simulink model "c00015M_harness"  (R2018a)
settings: Solver=FixedStepAuto  StartTime=0.0  StopTime=300  FixedStep=0.1  RelTol=1e-3
undefined symbols (not defined in the file): A1, hmax, PriorityTank, R1, R2, sigbuilder_block, TempThreshold
(part 1 of 33)
settings Model: Creator=aarrieta  LastModifiedBy=umarkiegi

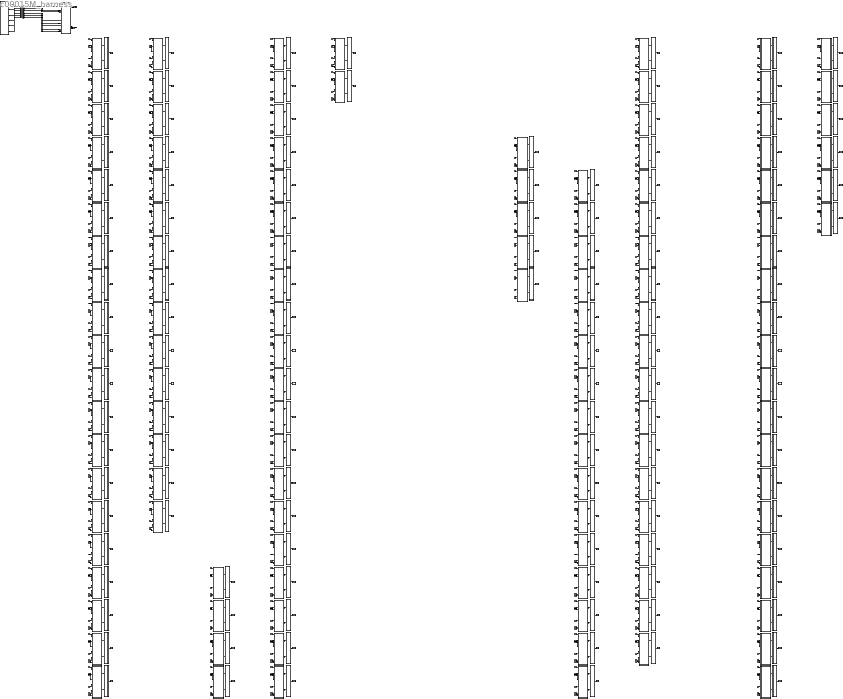
== system c00015M_harness ==
  CPSUT : Subsystem
  Eval : Subsystem
  Eval1 : Subsystem
  Eval10 : Subsystem
  Eval11 : Subsystem
  Eval12 : Subsystem
  Eval13 : Subsystem
  Eval14 : Subsystem
  Eval143 : Subsystem
  Eval144 : Subsystem
  Eval145 : Subsystem
  Eval146 : Subsystem
  Eval147 : Subsystem
  Eval15 : Subsystem
  Eval16 : Subsystem
  Eval164 : Subsystem
  Eval165 : Subsystem
  Eval166 : Subsystem
  Eval167 : Subsystem
  Eval168 : Subsystem
  Eval169 : Subsystem
  Eval17 : Subsystem
  Eval170 : Subsystem
  Eval171 : Subsystem
  Eval172 : Subsystem
  Eval173 : Subsystem
  Eval174 : Subsystem
  Eval175 : Subsystem
  Eval176 : Subsystem
  Eval177 : Subsystem
  Eval178 : Subsystem
  Eval179 : Subsystem
  Eval18 : Subsystem
  Eval180 : Subsystem
  Eval181 : Subsystem
  Eval182 : Subsystem
  Eval183 : Subsystem
  Eval184 : Subsystem
  Eval185 : Subsystem
  Eval186 : Subsystem
  Eval187 : Subsystem
  Eval188 : Subsystem
  Eval189 : Subsystem
  Eval19 : Subsystem
  Eval190 : Subsystem
  Eval191 : Subsystem
  Eval192 : Subsystem
  Eval193 : Subsystem
  Eval194 : Subsystem
  Eval195 : Subsystem
  Eval196 : Subsystem
  Eval197 : Subsystem
  Eval198 : Subsystem
  Eval2 : Subsystem
  Eval20 : Subsystem
  Eval21 : Subsystem
  Eval22 : Subsystem
  Eval220 : Subsystem
  Eval221 : Subsystem
  Eval222 : Subsystem
  Eval223 : Subsystem
  Eval224 : Subsystem
  Eval225 : Subsystem
  Eval226 : Subsystem
  Eval227 : Subsystem
  Eval228 : Subsystem
  Eval229 : Subsystem
  Eval23 : Subsystem
  Eval230 : Subsystem
  Eval231 : Subsystem
  Eval232 : Subsystem
  Eval233 : Subsystem
  Eval234 : Subsystem
  Eval235 : Subsystem
  Eval236 : Subsystem
  Eval237 : Subsystem
  Eval238 : Subsystem
  Eval239 : Subsystem
  Eval24 : Subsystem
  Eval240 : Subsystem
  Eval241 : Subsystem
  Eval242 : Subsystem
  Eval243 : Subsystem
  Eval244 : Subsystem
  Eval245 : Subsystem
  Eval25 : Subsystem
  Eval26 : Subsystem
  Eval27 : Subsystem
  Eval28 : Subsystem
  Eval29 : Subsystem
  Eval3 : Subsystem
  Eval30 : Subsystem
  Eval31 : Subsystem
  Eval32 : Subsystem
  Eval33 : Subsystem
  Eval34 : Subsystem
  Eval4 : Subsystem
  Eval5 : Subsystem
  Eval56 : Subsystem
  Eval57 : Subsystem
  Eval58 : Subsystem
  Eval59 : Subsystem
  Eval6 : Subsystem
  Eval60 : Subsystem
  Eval61 : Subsystem
  Eval62 : Subsystem
  Eval63 : Subsystem
  Eval64 : Subsystem
  Eval65 : Subsystem
  Eval66 : Subsystem
  Eval67 : Subsystem
  Eval68 : Subsystem
  Eval69 : Subsystem
  Eval7 : Subsystem
  Eval70 : Subsystem
  Eval71 : Subsystem
  Eval72 : Subsystem
  Eval73 : Subsystem
  Eval74 : Subsystem
  Eval75 : Subsystem
  Eval76 : Subsystem
  Eval77 : Subsystem
  Eval78 : Subsystem
  Eval79 : Subsystem
  Eval8 : Subsystem
  Eval80 : Subsystem
  Eval81 : Subsystem
  Eval9 : Subsystem
  Inputs : Subsystem  Tag=STV Subsys  LoadFcn=sigbuilder_block('load');  StartFcn=sigbuilder_block('start');  StopFcn=sigbuilder_block('stop');  ClipboardFcn=sigbuilder_block('clipboard');  mask(Sigbuilder block){tuvar=[0:10]}
      mask init:
      | if ~strcmp(get_param(bdroot(gcb),'SimulationStatus'),'stopped'),tuvar = sigbuilder_block('maskInit'); end
      settings: CopyFcn=sigbuilder_block('copy');  DeleteFcn=sigbuilder_block('delete');  ModelCloseFcn=sigbuilder_block('modelClose');  PreSaveFcn=sigbuilder_block('preSave');  PauseFcn=sigbuilder_block('pause');  ContinueFcn=sigbuilder_block('continue');  NameChangeFcn=sigbuilder_block('namechange');  OpenFcn=sigbuilder_block('open',[276.75 163.5 675.75 486.75 ]);  CloseFcn=sigbuilder_block('close');
      mask Display: plot(0, 0, 100, 100,[2, 2, 32, 32, 2], [68, 8, 8, 68, 68],[32, 2], [38, 38], [32, 19, 2],[53, 60, 44], [32, 17, 17, 2],[16, 16, 31, 31]);txt = getActiveGroup(gcbh);text(2, 100, txt,'verticalAlignment', 'top');
  M001 : Subsystem
  M002 : Subsystem
  M003 : Subsystem
  M004 : Subsystem
  M005 : Subsystem
  M006 : Subsystem
  M007 : Subsystem
  M008 : Subsystem
  M009 : Subsystem
  M010 : Subsystem
  M011 : Subsystem
  M012 : Subsystem
  M013 : Subsystem
  M014 : Subsystem
  M015 : Subsystem
  M016 : Subsystem
  M017 : Subsystem
  M018 : Subsystem
  M019 : Subsystem
  M020 : Subsystem
  M021 : Subsystem
  M022 : Subsystem
  M023 : Subsystem
  M024 : Subsystem
  M025 : Subsystem
  M026 : Subsystem
  M027 : Subsystem
  M028 : Subsystem
  M029 : Subsystem
  M030 : Subsystem
  M031 : Subsystem
  M032 : Subsystem
  M033 : Subsystem
  M034 : Subsystem
  M035 : Subsystem
  M057 : Subsystem
  M058 : Subsystem
  M059 : Subsystem
  M060 : Subsystem
  M061 : Subsystem
  M062 : Subsystem
  M063 : Subsystem
  M064 : Subsystem
  M065 : Subsystem
  M066 : Subsystem
  M067 : Subsystem
  M068 : Subsystem
  M069 : Subsystem
  M070 : Subsystem
  M071 : Subsystem
  M072 : Subsystem
  M073 : Subsystem
  M074 : Subsystem
  M075 : Subsystem
  M076 : Subsystem
  M077 : Subsystem
  M078 : Subsystem
  M079 : Subsystem
  M080 : Subsystem
  M081 : Subsystem
  M082 : Subsystem
  M144 : Subsystem
  M145 : Subsystem
  M146 : Subsystem
  M147 : Subsystem
  M148 : Subsystem
  M165 : Subsystem
  M166 : Subsystem
  M167 : Subsystem
  M168 : Subsystem
  M169 : Subsystem
  M170 : Subsystem
  M171 : Subsystem
  M172 : Subsystem
  M173 : Subsystem
  M174 : Subsystem
  M175 : Subsystem
  M176 : Subsystem
  M177 : Subsystem
  M178 : Subsystem
  M179 : Subsystem
  M180 : Subsystem
  M181 : Subsystem
  M182 : Subsystem
  M183 : Subsystem
  M184 : Subsystem
  M185 : Subsystem
  M186 : Subsystem
  M187 : Subsystem
  M188 : Subsystem
  M189 : Subsystem
  M190 : Subsystem
  M191 : Subsystem
  M192 : Subsystem
  M193 : Subsystem
  M194 : Subsystem
  M195 : Subsystem
  M196 : Subsystem
  M197 : Subsystem
  M198 : Subsystem
  M199 : Subsystem
  M221 : Subsystem
  M222 : Subsystem
  M223 : Subsystem
  M224 : Subsystem
  M225 : Subsystem
  M226 : Subsystem
  M227 : Subsystem
  M228 : Subsystem
  M229 : Subsystem
  M230 : Subsystem
  M231 : Subsystem
  M232 : Subsystem
  M233 : Subsystem
  M234 : Subsystem
  M235 : Subsystem
  M236 : Subsystem
  M237 : Subsystem
  M238 : Subsystem
  M239 : Subsystem
  M240 : Subsystem
  M241 : Subsystem
  M242 : Subsystem
  M243 : Subsystem
  M244 : Subsystem
  M245 : Subsystem
  M246 : Subsystem
  To Workspace : ToWorkspace  VariableName=mutant001  SampleTime=-1
  To Workspace1 : ToWorkspace  VariableName=mutant002  SampleTime=-1
  To Workspace10 : ToWorkspace  VariableName=mutant011  SampleTime=-1
  To Workspace11 : ToWorkspace  VariableName=mutant012  SampleTime=-1
  To Workspace12 : ToWorkspace  VariableName=mutant013  SampleTime=-1
  To Workspace13 : ToWorkspace  VariableName=mutant014  SampleTime=-1
  To Workspace14 : ToWorkspace  VariableName=mutant015  SampleTime=-1
  To Workspace143 : ToWorkspace  VariableName=mutant144  SampleTime=-1
  To Workspace144 : ToWorkspace  VariableName=mutant145  SampleTime=-1
  To Workspace145 : ToWorkspace  VariableName=mutant146  SampleTime=-1
  To Workspace146 : ToWorkspace  VariableName=mutant147  SampleTime=-1
  To Workspace147 : ToWorkspace  VariableName=mutant148  SampleTime=-1
  To Workspace15 : ToWorkspace  VariableName=mutant016  SampleTime=-1
  To Workspace16 : ToWorkspace  VariableName=mutant017  SampleTime=-1
  To Workspace164 : ToWorkspace  VariableName=mutant165  SampleTime=-1
  To Workspace165 : ToWorkspace  VariableName=mutant166  SampleTime=-1
  To Workspace166 : ToWorkspace  VariableName=mutant167  SampleTime=-1
  To Workspace167 : ToWorkspace  VariableName=mutant168  SampleTime=-1
  To Workspace168 : ToWorkspace  VariableName=mutant169  SampleTime=-1
  To Workspace169 : ToWorkspace  VariableName=mutant170  SampleTime=-1
  To Workspace17 : ToWorkspace  VariableName=mutant018  SampleTime=-1
  To Workspace170 : ToWorkspace  VariableName=mutant171  SampleTime=-1
  To Workspace171 : ToWorkspace  VariableName=mutant172  SampleTime=-1
  To Workspace172 : ToWorkspace  VariableName=mutant173  SampleTime=-1
  To Workspace173 : ToWorkspace  VariableName=mutant174  SampleTime=-1
  To Workspace174 : ToWorkspace  VariableName=mutant175  SampleTime=-1
  To Workspace175 : ToWorkspace  VariableName=mutant176  SampleTime=-1
  To Workspace176 : ToWorkspace  VariableName=mutant177  SampleTime=-1
  To Workspace177 : ToWorkspace  VariableName=mutant178  SampleTime=-1
  To Workspace178 : ToWorkspace  VariableName=mutant179  SampleTime=-1
  To Workspace179 : ToWorkspace  VariableName=mutant180  SampleTime=-1
  To Workspace18 : ToWorkspace  VariableName=mutant019  SampleTime=-1
  To Workspace180 : ToWorkspace  VariableName=mutant181  SampleTime=-1
  To Workspace181 : ToWorkspace  VariableName=mutant182  SampleTime=-1
  To Workspace182 : ToWorkspace  VariableName=mutant183  SampleTime=-1
  To Workspace183 : ToWorkspace  VariableName=mutant184  SampleTime=-1
  To Workspace184 : ToWorkspace  VariableName=mutant185  SampleTime=-1
  To Workspace185 : ToWorkspace  VariableName=mutant186  SampleTime=-1
  To Workspace186 : ToWorkspace  VariableName=mutant187  SampleTime=-1
  To Workspace187 : ToWorkspace  VariableName=mutant188  SampleTime=-1
  To Workspace188 : ToWorkspace  VariableName=mutant189  SampleTime=-1
  To Workspace189 : ToWorkspace  VariableName=mutant190  SampleTime=-1
  To Workspace19 : ToWorkspace  VariableName=mutant020  SampleTime=-1
  To Workspace190 : ToWorkspace  VariableName=mutant191  SampleTime=-1
  To Workspace191 : ToWorkspace  VariableName=mutant192  SampleTime=-1
  To Workspace192 : ToWorkspace  VariableName=mutant193  SampleTime=-1
  To Workspace193 : ToWorkspace  VariableName=mutant194  SampleTime=-1
  To Workspace194 : ToWorkspace  VariableName=mutant195  SampleTime=-1
  To Workspace195 : ToWorkspace  VariableName=mutant196  SampleTime=-1
  To Workspace196 : ToWorkspace  VariableName=mutant197  SampleTime=-1
  To Workspace197 : ToWorkspace  VariableName=mutant198  SampleTime=-1
  To Workspace198 : ToWorkspace  VariableName=mutant199  SampleTime=-1
  To Workspace2 : ToWorkspace  VariableName=mutant003  SampleTime=-1
  To Workspace20 : ToWorkspace  VariableName=mutant021  SampleTime=-1
  To Workspace21 : ToWorkspace  VariableName=mutant022  SampleTime=-1
  To Workspace22 : ToWorkspace  VariableName=mutant023  SampleTime=-1
  To Workspace220 : ToWorkspace  VariableName=mutant221  SampleTime=-1
  To Workspace221 : ToWorkspace  VariableName=mutant222  SampleTime=-1
  To Workspace222 : ToWorkspace  VariableName=mutant223  SampleTime=-1
  To Workspace223 : ToWorkspace  VariableName=mutant224  SampleTime=-1
  To Workspace224 : ToWorkspace  VariableName=mutant225  SampleTime=-1
  To Workspace225 : ToWorkspace  VariableName=mutant226  SampleTime=-1
  To Workspace226 : ToWorkspace  VariableName=mutant227  SampleTime=-1
  To Workspace227 : ToWorkspace  VariableName=mutant228  SampleTime=-1
  To Workspace228 : ToWorkspace  VariableName=mutant229  SampleTime=-1
  To Workspace229 : ToWorkspace  VariableName=mutant230  SampleTime=-1
  To Workspace23 : ToWorkspace  VariableName=mutant024  SampleTime=-1
  To Workspace230 : ToWorkspace  VariableName=mutant231  SampleTime=-1
  To Workspace231 : ToWorkspace  VariableName=mutant232  SampleTime=-1
  To Workspace232 : ToWorkspace  VariableName=mutant233  SampleTime=-1
  To Workspace233 : ToWorkspace  VariableName=mutant234  SampleTime=-1
  To Workspace234 : ToWorkspace  VariableName=mutant235  SampleTime=-1
  To Workspace235 : ToWorkspace  VariableName=mutant236  SampleTime=-1
  To Workspace236 : ToWorkspace  VariableName=mutant237  SampleTime=-1
  To Workspace237 : ToWorkspace  VariableName=mutant238  SampleTime=-1
  To Workspace238 : ToWorkspace  VariableName=mutant239  SampleTime=-1
  To Workspace239 : ToWorkspace  VariableName=mutant240  SampleTime=-1
  To Workspace24 : ToWorkspace  VariableName=mutant025  SampleTime=-1
  To Workspace240 : ToWorkspace  VariableName=mutant241  SampleTime=-1
  To Workspace241 : ToWorkspace  VariableName=mutant242  SampleTime=-1
  To Workspace242 : ToWorkspace  VariableName=mutant243  SampleTime=-1
  To Workspace243 : ToWorkspace  VariableName=mutant244  SampleTime=-1
  To Workspace244 : ToWorkspace  VariableName=mutant245  SampleTime=-1
  To Workspace245 : ToWorkspace  VariableName=mutant246  SampleTime=-1
  To Workspace25 : ToWorkspace  VariableName=mutant026  SampleTime=-1
  To Workspace26 : ToWorkspace  VariableName=mutant027  SampleTime=-1
  To Workspace27 : ToWorkspace  VariableName=mutant028  SampleTime=-1
  To Workspace28 : ToWorkspace  VariableName=mutant029  SampleTime=-1
  To Workspace29 : ToWorkspace  VariableName=mutant030  SampleTime=-1
  To Workspace3 : ToWorkspace  VariableName=mutant004  SampleTime=-1
  To Workspace30 : ToWorkspace  VariableName=mutant031  SampleTime=-1
  To Workspace31 : ToWorkspace  VariableName=mutant032  SampleTime=-1
  To Workspace32 : ToWorkspace  VariableName=mutant033  SampleTime=-1
  To Workspace33 : ToWorkspace  VariableName=mutant034  SampleTime=-1
  To Workspace34 : ToWorkspace  VariableName=mutant035  SampleTime=-1
  To Workspace4 : ToWorkspace  VariableName=mutant005  SampleTime=-1
  To Workspace5 : ToWorkspace  VariableName=mutant006  SampleTime=-1
  To Workspace56 : ToWorkspace  VariableName=mutant057  SampleTime=-1
  To Workspace57 : ToWorkspace  VariableName=mutant058  SampleTime=-1
  To Workspace58 : ToWorkspace  VariableName=mutant059  SampleTime=-1
  To Workspace59 : ToWorkspace  VariableName=mutant060  SampleTime=-1
  To Workspace6 : ToWorkspace  VariableName=mutant007  SampleTime=-1
  To Workspace60 : ToWorkspace  VariableName=mutant061  SampleTime=-1
  To Workspace61 : ToWorkspace  VariableName=mutant062  SampleTime=-1
  To Workspace62 : ToWorkspace  VariableName=mutant063  SampleTime=-1
  To Workspace63 : ToWorkspace  VariableName=mutant064  SampleTime=-1
  To Workspace64 : ToWorkspace  VariableName=mutant065  SampleTime=-1
  To Workspace65 : ToWorkspace  VariableName=mutant066  SampleTime=-1
  To Workspace66 : ToWorkspace  VariableName=mutant067  SampleTime=-1
  To Workspace67 : ToWorkspace  VariableName=mutant068  SampleTime=-1
  To Workspace68 : ToWorkspace  VariableName=mutant069  SampleTime=-1
  To Workspace69 : ToWorkspace  VariableName=mutant070  SampleTime=-1
  To Workspace7 : ToWorkspace  VariableName=mutant008  SampleTime=-1
  To Workspace70 : ToWorkspace  VariableName=mutant071  SampleTime=-1
  To Workspace71 : ToWorkspace  VariableName=mutant072  SampleTime=-1
  To Workspace72 : ToWorkspace  VariableName=mutant073  SampleTime=-1
  To Workspace73 : ToWorkspace  VariableName=mutant074  SampleTime=-1
  To Workspace74 : ToWorkspace  VariableName=mutant075  SampleTime=-1
  To Workspace75 : ToWorkspace  VariableName=mutant076  SampleTime=-1
  To Workspace76 : ToWorkspace  VariableName=mutant077  SampleTime=-1
  To Workspace77 : ToWorkspace  VariableName=mutant078  SampleTime=-1
  To Workspace78 : ToWorkspace  VariableName=mutant079  SampleTime=-1
  To Workspace79 : ToWorkspace  VariableName=mutant080  SampleTime=-1
  To Workspace8 : ToWorkspace  VariableName=mutant009  SampleTime=-1
  To Workspace80 : ToWorkspace  VariableName=mutant081  SampleTime=-1
  To Workspace81 : ToWorkspace  VariableName=mutant082  SampleTime=-1
  To Workspace9 : ToWorkspace  VariableName=mutant010  SampleTime=-1
  dtc_CT1 : DataTypeConversion
  dtc_CT3 : DataTypeConversion
  dtc_EB1 : DataTypeConversion
  dtc_EB3 : DataTypeConversion
  dtc_T1 : DataTypeConversion
  dtc_T3 : DataTypeConversion
  LL1 : Outport
  LL3 : Outport  Port=2
  tag scope: out1=global, out3=global
  wires:
  CPSUT/1(LL1) -> [out1], LL1/1
  CPSUT/2(LL3) -> [out3], LL3/1
  [in1] -> M001/1(CT1)
  [in5] -> M001/2(T1)
  [in6] -> M001/3(EB1)
  [in13] -> M001/4(CT3)
  [in17] -> M001/5(T3)
  [in18] -> M001/6(EB3)
  Eval/1(Out1) -> To Workspace/1
  M001/1(LL1) -> Eval/1(In1)
  M001/2(LL3) -> Eval/2(In3)
  [in1] -> M002/1(CT1)
  [in5] -> M002/2(T1)
  [in6] -> M002/3(EB1)
  [in13] -> M002/4(CT3)
  [in17] -> M002/5(T3)
  [in18] -> M002/6(EB3)
  M002/1(LL1) -> Eval1/1(In1)
  M002/2(LL3) -> Eval1/2(In3)
  Eval1/1(Out1) -> To Workspace1/1
  [in1] -> M003/1(CT1)
  [in5] -> M003/2(T1)
  [in6] -> M003/3(EB1)
  [in13] -> M003/4(CT3)
  [in17] -> M003/5(T3)
  [in18] -> M003/6(EB3)
  M003/1(LL1) -> Eval2/1(In1)
  M003/2(LL3) -> Eval2/2(In3)
  Eval2/1(Out1) -> To Workspace2/1
  [in1] -> M004/1(CT1)
  [in5] -> M004/2(T1)
  [in6] -> M004/3(EB1)
  [in13] -> M004/4(CT3)
  [in17] -> M004/5(T3)
  [in18] -> M004/6(EB3)
  M004/1(LL1) -> Eval3/1(In1)
  M004/2(LL3) -> Eval3/2(In3)
  Eval3/1(Out1) -> To Workspace3/1
  [in1] -> M005/1(CT1)
  [in5] -> M005/2(T1)
  [in6] -> M005/3(EB1)
  [in13] -> M005/4(CT3)
  [in17] -> M005/5(T3)
  [in18] -> M005/6(EB3)
  M005/1(LL1) -> Eval4/1(In1)
  M005/2(LL3) -> Eval4/2(In3)
  Eval4/1(Out1) -> To Workspace4/1
  [in1] -> M006/1(CT1)
  [in5] -> M006/2(T1)
  [in6] -> M006/3(EB1)
  [in13] -> M006/4(CT3)
  [in17] -> M006/5(T3)
  [in18] -> M006/6(EB3)
  M006/1(LL1) -> Eval5/1(In1)
  M006/2(LL3) -> Eval5/2(In3)
  Eval5/1(Out1) -> To Workspace5/1
  [in1] -> M007/1(CT1)
  [in5] -> M007/2(T1)
  [in6] -> M007/3(EB1)
  [in13] -> M007/4(CT3)
  [in17] -> M007/5(T3)
  [in18] -> M007/6(EB3)
  M007/1(LL1) -> Eval6/1(In1)
  M007/2(LL3) -> Eval6/2(In3)
  Eval6/1(Out1) -> To Workspace6/1
  [in1] -> M008/1(CT1)
  [in5] -> M008/2(T1)
  [in6] -> M008/3(EB1)
  [in13] -> M008/4(CT3)
  [in17] -> M008/5(T3)
  [in18] -> M008/6(EB3)
  M008/1(LL1) -> Eval7/1(In1)
  M008/2(LL3) -> Eval7/2(In3)
  Eval7/1(Out1) -> To Workspace7/1
  [in1] -> M009/1(CT1)
  [in5] -> M009/2(T1)
  [in6] -> M009/3(EB1)
  [in13] -> M009/4(CT3)
  [in17] -> M009/5(T3)
  [in18] -> M009/6(EB3)
  M009/1(LL1) -> Eval8/1(In1)
  M009/2(LL3) -> Eval8/2(In3)
  Eval8/1(Out1) -> To Workspace8/1
  [in1] -> M010/1(CT1)
  [in5] -> M010/2(T1)
  [in6] -> M010/3(EB1)
  [in13] -> M010/4(CT3)
  [in17] -> M010/5(T3)
  [in18] -> M010/6(EB3)
  M010/1(LL1) -> Eval9/1(In1)
  M010/2(LL3) -> Eval9/2(In3)
  Eval9/1(Out1) -> To Workspace9/1
  [in1] -> M011/1(CT1)
  [in5] -> M011/2(T1)
  [in6] -> M011/3(EB1)
  [in13] -> M011/4(CT3)
  [in17] -> M011/5(T3)
  [in18] -> M011/6(EB3)
  M011/1(LL1) -> Eval10/1(In1)
  M011/2(LL3) -> Eval10/2(In3)
  Eval10/1(Out1) -> To Workspace10/1
  [in1] -> M012/1(CT1)
  [in5] -> M012/2(T1)
  [in6] -> M012/3(EB1)
  [in13] -> M012/4(CT3)
  [in17] -> M012/5(T3)
  [in18] -> M012/6(EB3)
  M012/1(LL1) -> Eval11/1(In1)
  M012/2(LL3) -> Eval11/2(In3)
  Eval11/1(Out1) -> To Workspace11/1
  [in1] -> M013/1(CT1)
  [in5] -> M013/2(T1)
  [in6] -> M013/3(EB1)
  [in13] -> M013/4(CT3)
  [in17] -> M013/5(T3)
  [in18] -> M013/6(EB3)
  M013/1(LL1) -> Eval12/1(In1)
  M013/2(LL3) -> Eval12/2(In3)
  Eval12/1(Out1) -> To Workspace12/1
  [in1] -> M014/1(CT1)
  [in5] -> M014/2(T1)
  [in6] -> M014/3(EB1)
  [in13] -> M014/4(CT3)
  [in17] -> M014/5(T3)
  [in18] -> M014/6(EB3)
  M014/1(LL1) -> Eval13/1(In1)
  M014/2(LL3) -> Eval13/2(In3)
  Eval13/1(Out1) -> To Workspace13/1
  [in1] -> M015/1(CT1)
  [in5] -> M015/2(T1)
  [in6] -> M015/3(EB1)
  [in13] -> M015/4(CT3)
  [in17] -> M015/5(T3)
  [in18] -> M015/6(EB3)
  M015/1(LL1) -> Eval14/1(In1)
  M015/2(LL3) -> Eval14/2(In3)
  Eval14/1(Out1) -> To Workspace14/1
  [in1] -> M016/1(CT1)
  [in5] -> M016/2(T1)
  [in6] -> M016/3(EB1)
  [in13] -> M016/4(CT3)
  [in17] -> M016/5(T3)
  [in18] -> M016/6(EB3)
  M016/1(LL1) -> Eval15/1(In1)
  M016/2(LL3) -> Eval15/2(In3)
  Eval15/1(Out1) -> To Workspace15/1
  [in1] -> M017/1(CT1)
  [in5] -> M017/2(T1)
  [in6] -> M017/3(EB1)
  [in13] -> M017/4(CT3)
  [in17] -> M017/5(T3)
  [in18] -> M017/6(EB3)
  M017/1(LL1) -> Eval16/1(In1)
  M017/2(LL3) -> Eval16/2(In3)
  Eval16/1(Out1) -> To Workspace16/1
  [in1] -> M018/1(CT1)
  [in5] -> M018/2(T1)
  [in6] -> M018/3(EB1)
  [in13] -> M018/4(CT3)
  [in17] -> M018/5(T3)
  [in18] -> M018/6(EB3)
  M018/1(LL1) -> Eval17/1(In1)
  M018/2(LL3) -> Eval17/2(In3)
  Eval17/1(Out1) -> To Workspace17/1
  [in1] -> M019/1(CT1)
  [in5] -> M019/2(T1)
  [in6] -> M019/3(EB1)
  [in13] -> M019/4(CT3)
  [in17] -> M019/5(T3)
  [in18] -> M019/6(EB3)
  M019/1(LL1) -> Eval18/1(In1)
  M019/2(LL3) -> Eval18/2(In3)
  Eval18/1(Out1) -> To Workspace18/1
  [in1] -> M020/1(CT1)
  [in5] -> M020/2(T1)
  [in6] -> M020/3(EB1)
  [in13] -> M020/4(CT3)
  [in17] -> M020/5(T3)
  [in18] -> M020/6(EB3)
  M020/1(LL1) -> Eval19/1(In1)
  M020/2(LL3) -> Eval19/2(In3)
  Eval19/1(Out1) -> To Workspace19/1
  [in1] -> M021/1(CT1)
  [in5] -> M021/2(T1)
  [in6] -> M021/3(EB1)
  [in13] -> M021/4(CT3)
  [in17] -> M021/5(T3)
  [in18] -> M021/6(EB3)
  M021/1(LL1) -> Eval20/1(In1)
  M021/2(LL3) -> Eval20/2(In3)
  Eval20/1(Out1) -> To Workspace20/1
  [in1] -> M022/1(CT1)
  [in5] -> M022/2(T1)
  [in6] -> M022/3(EB1)
  [in13] -> M022/4(CT3)
  [in17] -> M022/5(T3)
  [in18] -> M022/6(EB3)
  M022/1(LL1) -> Eval21/1(In1)
  M022/2(LL3) -> Eval21/2(In3)
  Eval21/1(Out1) -> To Workspace21/1
  [in1] -> M023/1(CT1)
  [in5] -> M023/2(T1)
  [in6] -> M023/3(EB1)
  [in13] -> M023/4(CT3)
  [in17] -> M023/5(T3)
  [in18] -> M023/6(EB3)
  M023/1(LL1) -> Eval22/1(In1)
  M023/2(LL3) -> Eval22/2(In3)
  Eval22/1(Out1) -> To Workspace22/1
  [in1] -> M024/1(CT1)
  [in5] -> M024/2(T1)
  [in6] -> M024/3(EB1)
  [in13] -> M024/4(CT3)
  [in17] -> M024/5(T3)
  [in18] -> M024/6(EB3)
  M024/1(LL1) -> Eval23/1(In1)
  M024/2(LL3) -> Eval23/2(In3)
  Eval23/1(Out1) -> To Workspace23/1
  [in1] -> M025/1(CT1)
  [in5] -> M025/2(T1)
  [in6] -> M025/3(EB1)
  [in13] -> M025/4(CT3)
  [in17] -> M025/5(T3)
  [in18] -> M025/6(EB3)
  M025/1(LL1) -> Eval24/1(In1)
  M025/2(LL3) -> Eval24/2(In3)
  Eval24/1(Out1) -> To Workspace24/1
  [in1] -> M026/1(CT1)
  [in5] -> M026/2(T1)
  [in6] -> M026/3(EB1)
  [in13] -> M026/4(CT3)
  [in17] -> M026/5(T3)
  [in18] -> M026/6(EB3)
  M026/1(LL1) -> Eval25/1(In1)
  M026/2(LL3) -> Eval25/2(In3)
  Eval25/1(Out1) -> To Workspace25/1
  [in1] -> M027/1(CT1)
  [in5] -> M027/2(T1)
  [in6] -> M027/3(EB1)
  [in13] -> M027/4(CT3)
  [in17] -> M027/5(T3)
  [in18] -> M027/6(EB3)
  M027/1(LL1) -> Eval26/1(In1)
  M027/2(LL3) -> Eval26/2(In3)
  Eval26/1(Out1) -> To Workspace26/1
  [in1] -> M028/1(CT1)
  [in5] -> M028/2(T1)
  [in6] -> M028/3(EB1)
  [in13] -> M028/4(CT3)
  [in17] -> M028/5(T3)
  [in18] -> M028/6(EB3)
  M028/1(LL1) -> Eval27/1(In1)
  M028/2(LL3) -> Eval27/2(In3)
  Eval27/1(Out1) -> To Workspace27/1
  [in1] -> M029/1(CT1)
  [in5] -> M029/2(T1)
  [in6] -> M029/3(EB1)
  [in13] -> M029/4(CT3)
  [in17] -> M029/5(T3)
  [in18] -> M029/6(EB3)
  M029/1(LL1) -> Eval28/1(In1)
  M029/2(LL3) -> Eval28/2(In3)
  Eval28/1(Out1) -> To Workspace28/1
  [in1] -> M030/1(CT1)
  [in5] -> M030/2(T1)
  [in6] -> M030/3(EB1)
  [in13] -> M030/4(CT3)
  [in17] -> M030/5(T3)
  [in18] -> M030/6(EB3)
  M030/1(LL1) -> Eval29/1(In1)
  M030/2(LL3) -> Eval29/2(In3)
  Eval29/1(Out1) -> To Workspace29/1
  [in1] -> M031/1(CT1)
  [in5] -> M031/2(T1)
  [in6] -> M031/3(EB1)
  [in13] -> M031/4(CT3)
  [in17] -> M031/5(T3)
  [in18] -> M031/6(EB3)
  M031/1(LL1) -> Eval30/1(In1)
  M031/2(LL3) -> Eval30/2(In3)
  Eval30/1(Out1) -> To Workspace30/1
  [in1] -> M032/1(CT1)
  [in5] -> M032/2(T1)
  [in6] -> M032/3(EB1)
  [in13] -> M032/4(CT3)
  [in17] -> M032/5(T3)
  [in18] -> M032/6(EB3)
  M032/1(LL1) -> Eval31/1(In1)
  M032/2(LL3) -> Eval31/2(In3)
  Eval31/1(Out1) -> To Workspace31/1
  [in1] -> M033/1(CT1)
  [in5] -> M033/2(T1)
  [in6] -> M033/3(EB1)
  [in13] -> M033/4(CT3)
  [in17] -> M033/5(T3)
  [in18] -> M033/6(EB3)
  M033/1(LL1) -> Eval32/1(In1)
  M033/2(LL3) -> Eval32/2(In3)
  Eval32/1(Out1) -> To Workspace32/1
  [in1] -> M034/1(CT1)
  [in5] -> M034/2(T1)
  [in6] -> M034/3(EB1)
  [in13] -> M034/4(CT3)
  [in17] -> M034/5(T3)
  [in18] -> M034/6(EB3)
  M034/1(LL1) -> Eval33/1(In1)
  M034/2(LL3) -> Eval33/2(In3)
  Eval33/1(Out1) -> To Workspace33/1
  [in1] -> M035/1(CT1)
  [in5] -> M035/2(T1)
  [in6] -> M035/3(EB1)
  [in13] -> M035/4(CT3)
  [in17] -> M035/5(T3)
  [in18] -> M035/6(EB3)
  M035/1(LL1) -> Eval34/1(In1)
  M035/2(LL3) -> Eval34/2(In3)
  Eval34/1(Out1) -> To Workspace34/1
  [in1] -> M057/1(CT1)
  [in5] -> M057/2(T1)
  [in6] -> M057/3(EB1)
  [in13] -> M057/4(CT3)
  [in17] -> M057/5(T3)
  [in18] -> M057/6(EB3)
  M057/1(LL1) -> Eval56/1(In1)
  M057/2(LL3) -> Eval56/2(In3)
  Eval56/1(Out1) -> To Workspace56/1
  [in1] -> M058/1(CT1)
  [in5] -> M058/2(T1)
  [in6] -> M058/3(EB1)
  [in13] -> M058/4(CT3)
  [in17] -> M058/5(T3)
  [in18] -> M058/6(EB3)
  M058/1(LL1) -> Eval57/1(In1)
  M058/2(LL3) -> Eval57/2(In3)
  Eval57/1(Out1) -> To Workspace57/1
  [in1] -> M059/1(CT1)
  [in5] -> M059/2(T1)
  [in6] -> M059/3(EB1)
  [in13] -> M059/4(CT3)
  [in17] -> M059/5(T3)
  [in18] -> M059/6(EB3)
  M059/1(LL1) -> Eval58/1(In1)
  M059/2(LL3) -> Eval58/2(In3)
  Eval58/1(Out1) -> To Workspace58/1
  [in1] -> M060/1(CT1)
  [in5] -> M060/2(T1)
  [in6] -> M060/3(EB1)
  [in13] -> M060/4(CT3)
  [in17] -> M060/5(T3)
  [in18] -> M060/6(EB3)
  M060/1(LL1) -> Eval59/1(In1)
  M060/2(LL3) -> Eval59/2(In3)
  Eval59/1(Out1) -> To Workspace59/1
  [in1] -> M061/1(CT1)
  [in5] -> M061/2(T1)
  [in6] -> M061/3(EB1)
  [in13] -> M061/4(CT3)
  [in17] -> M061/5(T3)
  [in18] -> M061/6(EB3)
  M061/1(LL1) -> Eval60/1(In1)
  M061/2(LL3) -> Eval60/2(In3)
  Eval60/1(Out1) -> To Workspace60/1
  [in1] -> M062/1(CT1)
  [in5] -> M062/2(T1)
  [in6] -> M062/3(EB1)
  [in13] -> M062/4(CT3)
  [in17] -> M062/5(T3)
  [in18] -> M062/6(EB3)
  M062/1(LL1) -> Eval61/1(In1)
  M062/2(LL3) -> Eval61/2(In3)
  Eval61/1(Out1) -> To Workspace61/1
  [in1] -> M063/1(CT1)
  [in5] -> M063/2(T1)
  [in6] -> M063/3(EB1)
  [in13] -> M063/4(CT3)
  [in17] -> M063/5(T3)
  [in18] -> M063/6(EB3)
  M063/1(LL1) -> Eval62/1(In1)
  M063/2(LL3) -> Eval62/2(In3)
  Eval62/1(Out1) -> To Workspace62/1
  [in1] -> M064/1(CT1)
  [in5] -> M064/2(T1)
  [in6] -> M064/3(EB1)
  [in13] -> M064/4(CT3)
  [in17] -> M064/5(T3)
  [in18] -> M064/6(EB3)
  M064/1(LL1) -> Eval63/1(In1)
  M064/2(LL3) -> Eval63/2(In3)
  Eval63/1(Out1) -> To Workspace63/1
  [in1] -> M065/1(CT1)
  [in5] -> M065/2(T1)
  [in6] -> M065/3(EB1)
  [in13] -> M065/4(CT3)
  [in17] -> M065/5(T3)
  [in18] -> M065/6(EB3)
  M065/1(LL1) -> Eval64/1(In1)
  M065/2(LL3) -> Eval64/2(In3)
  Eval64/1(Out1) -> To Workspace64/1
  [in1] -> M066/1(CT1)
  [in5] -> M066/2(T1)
  [in6] -> M066/3(EB1)
  [in13] -> M066/4(CT3)
  [in17] -> M066/5(T3)
  [in18] -> M066/6(EB3)
  M066/1(LL1) -> Eval65/1(In1)
  M066/2(LL3) -> Eval65/2(In3)
  Eval65/1(Out1) -> To Workspace65/1
  [in1] -> M067/1(CT1)
  [in5] -> M067/2(T1)
  [in6] -> M067/3(EB1)
  [in13] -> M067/4(CT3)
  [in17] -> M067/5(T3)
  [in18] -> M067/6(EB3)
  M067/1(LL1) -> Eval66/1(In1)
  M067/2(LL3) -> Eval66/2(In3)
  Eval66/1(Out1) -> To Workspace66/1
  [in1] -> M068/1(CT1)
  [in5] -> M068/2(T1)
  [in6] -> M068/3(EB1)
  [in13] -> M068/4(CT3)
  [in17] -> M068/5(T3)
  [in18] -> M068/6(EB3)
  M068/1(LL1) -> Eval67/1(In1)
  M068/2(LL3) -> Eval67/2(In3)
  Eval67/1(Out1) -> To Workspace67/1
  [in1] -> M069/1(CT1)
  [in5] -> M069/2(T1)
  [in6] -> M069/3(EB1)
  [in13] -> M069/4(CT3)
  [in17] -> M069/5(T3)
  [in18] -> M069/6(EB3)
  M069/1(LL1) -> Eval68/1(In1)
  M069/2(LL3) -> Eval68/2(In3)
  Eval68/1(Out1) -> To Workspace68/1
  [in1] -> M070/1(CT1)
  [in5] -> M070/2(T1)
  [in6] -> M070/3(EB1)
  [in13] -> M070/4(CT3)
  [in17] -> M070/5(T3)
  [in18] -> M070/6(EB3)
  M070/1(LL1) -> Eval69/1(In1)
  M070/2(LL3) -> Eval69/2(In3)
  Eval69/1(Out1) -> To Workspace69/1
  [in1] -> M071/1(CT1)
  [in5] -> M071/2(T1)
  [in6] -> M071/3(EB1)
  [in13] -> M071/4(CT3)
  [in17] -> M071/5(T3)
  [in18] -> M071/6(EB3)
  M071/1(LL1) -> Eval70/1(In1)
  M071/2(LL3) -> Eval70/2(In3)
  Eval70/1(Out1) -> To Workspace70/1
  [in1] -> M072/1(CT1)
  [in5] -> M072/2(T1)
  [in6] -> M072/3(EB1)
  [in13] -> M072/4(CT3)
  [in17] -> M072/5(T3)
  [in18] -> M072/6(EB3)
  M072/1(LL1) -> Eval71/1(In1)
  M072/2(LL3) -> Eval71/2(In3)
  Eval71/1(Out1) -> To Workspace71/1
  [in1] -> M073/1(CT1)
  [in5] -> M073/2(T1)
  [in6] -> M073/3(EB1)
  [in13] -> M073/4(CT3)
  [in17] -> M073/5(T3)
  [in18] -> M073/6(EB3)
  M073/1(LL1) -> Eval72/1(In1)
  M073/2(LL3) -> Eval72/2(In3)
  Eval72/1(Out1) -> To Workspace72/1
  [in1] -> M074/1(CT1)
  [in5] -> M074/2(T1)
  [in6] -> M074/3(EB1)
  [in13] -> M074/4(CT3)
  [in17] -> M074/5(T3)
  [in18] -> M074/6(EB3)
  M074/1(LL1) -> Eval73/1(In1)
  M074/2(LL3) -> Eval73/2(In3)
  Eval73/1(Out1) -> To Workspace73/1
  [in1] -> M075/1(CT1)
  [in5] -> M075/2(T1)
  [in6] -> M075/3(EB1)
  [in13] -> M075/4(CT3)
  [in17] -> M075/5(T3)
  [in18] -> M075/6(EB3)
  M075/1(LL1) -> Eval74/1(In1)
  M075/2(LL3) -> Eval74/2(In3)
  Eval74/1(Out1) -> To Workspace74/1
  [in1] -> M076/1(CT1)
  [in5] -> M076/2(T1)
  [in6] -> M076/3(EB1)
  [in13] -> M076/4(CT3)
  [in17] -> M076/5(T3)
  [in18] -> M076/6(EB3)
  M076/1(LL1) -> Eval75/1(In1)
  M076/2(LL3) -> Eval75/2(In3)
  Eval75/1(Out1) -> To Workspace75/1
  [in1] -> M077/1(CT1)
  [in5] -> M077/2(T1)
  [in6] -> M077/3(EB1)
  [in13] -> M077/4(CT3)
  [in17] -> M077/5(T3)
  [in18] -> M077/6(EB3)
  M077/1(LL1) -> Eval76/1(In1)
  M077/2(LL3) -> Eval76/2(In3)
  Eval76/1(Out1) -> To Workspace76/1
  [in1] -> M078/1(CT1)
  [in5] -> M078/2(T1)
  [in6] -> M078/3(EB1)
  [in13] -> M078/4(CT3)
  [in17] -> M078/5(T3)
  [in18] -> M078/6(EB3)
  M078/1(LL1) -> Eval77/1(In1)
  M078/2(LL3) -> Eval77/2(In3)
  Eval77/1(Out1) -> To Workspace77/1
  [in1] -> M079/1(CT1)
  [in5] -> M079/2(T1)
  [in6] -> M079/3(EB1)
  [in13] -> M079/4(CT3)
  [in17] -> M079/5(T3)
  [in18] -> M079/6(EB3)
  M079/1(LL1) -> Eval78/1(In1)
  M079/2(LL3) -> Eval78/2(In3)
  Eval78/1(Out1) -> To Workspace78/1
  [in1] -> M080/1(CT1)
  [in5] -> M080/2(T1)
  [in6] -> M080/3(EB1)
  [in13] -> M080/4(CT3)
  [in17] -> M080/5(T3)
  [in18] -> M080/6(EB3)
  M080/1(LL1) -> Eval79/1(In1)
  M080/2(LL3) -> Eval79/2(In3)
  Eval79/1(Out1) -> To Workspace79/1
  [in1] -> M081/1(CT1)
  [in5] -> M081/2(T1)
  [in6] -> M081/3(EB1)
  [in13] -> M081/4(CT3)
  [in17] -> M081/5(T3)
  [in18] -> M081/6(EB3)
  M081/1(LL1) -> Eval80/1(In1)
  M081/2(LL3) -> Eval80/2(In3)
  Eval80/1(Out1) -> To Workspace80/1
  [in1] -> M082/1(CT1)
  [in5] -> M082/2(T1)
  [in6] -> M082/3(EB1)
  [in13] -> M082/4(CT3)
  [in17] -> M082/5(T3)
  [in18] -> M082/6(EB3)
  M082/1(LL1) -> Eval81/1(In1)
  M082/2(LL3) -> Eval81/2(In3)
  Eval81/1(Out1) -> To Workspace81/1
  [in1] -> M144/1(CT1)
  [in5] -> M144/2(T1)
  [in6] -> M144/3(EB1)
  [in13] -> M144/4(CT3)
  [in17] -> M144/5(T3)
  [in18] -> M144/6(EB3)
  M144/1(LL1) -> Eval143/1(In1)
  M144/2(LL3) -> Eval143/2(In3)
  Eval143/1(Out1) -> To Workspace143/1
  [in1] -> M145/1(CT1)
  [in5] -> M145/2(T1)
  [in6] -> M145/3(EB1)
  [in13] -> M145/4(CT3)
  [in17] -> M145/5(T3)
  [in18] -> M145/6(EB3)
  M145/1(LL1) -> Eval144/1(In1)
  M145/2(LL3) -> Eval144/2(In3)
  Eval144/1(Out1) -> To Workspace144/1
  [in1] -> M146/1(CT1)
  [in5] -> M146/2(T1)
  [in6] -> M146/3(EB1)
  [in13] -> M146/4(CT3)
  [in17] -> M146/5(T3)
  [in18] -> M146/6(EB3)
  M146/1(LL1) -> Eval145/1(In1)
  M146/2(LL3) -> Eval145/2(In3)
  Eval145/1(Out1) -> To Workspace145/1
  [in1] -> M147/1(CT1)
  [in5] -> M147/2(T1)
  [in6] -> M147/3(EB1)
  [in13] -> M147/4(CT3)
  [in17] -> M147/5(T3)
  [in18] -> M147/6(EB3)
  M147/1(LL1) -> Eval146/1(In1)
  M147/2(LL3) -> Eval146/2(In3)
  Eval146/1(Out1) -> To Workspace146/1
  [in1] -> M148/1(CT1)
  [in5] -> M148/2(T1)
  [in6] -> M148/3(EB1)
  [in13] -> M148/4(CT3)
  [in17] -> M148/5(T3)
  [in18] -> M148/6(EB3)
  M148/1(LL1) -> Eval147/1(In1)
  M148/2(LL3) -> Eval147/2(In3)
  Eval147/1(Out1) -> To Workspace147/1
  [in1] -> M165/1(CT1)
  [in5] -> M165/2(T1)
  [in6] -> M165/3(EB1)
  [in13] -> M165/4(CT3)
  [in17] -> M165/5(T3)
  [in18] -> M165/6(EB3)
  M165/1(LL1) -> Eval164/1(In1)
  M165/2(LL3) -> Eval164/2(In3)
  Eval164/1(Out1) -> To Workspace164/1
  [in1] -> M166/1(CT1)
  [in5] -> M166/2(T1)
  [in6] -> M166/3(EB1)
  [in13] -> M166/4(CT3)
  [in17] -> M166/5(T3)
  [in18] -> M166/6(EB3)
  M166/1(LL1) -> Eval165/1(In1)
  M166/2(LL3) -> Eval165/2(In3)
  Eval165/1(Out1) -> To Workspace165/1
  [in1] -> M167/1(CT1)
  [in5] -> M167/2(T1)
  [in6] -> M167/3(EB1)
  [in13] -> M167/4(CT3)
  [in17] -> M167/5(T3)
  [in18] -> M167/6(EB3)
  M167/1(LL1) -> Eval166/1(In1)
  M167/2(LL3) -> Eval166/2(In3)
  Eval166/1(Out1) -> To Workspace166/1
  [in1] -> M168/1(CT1)
  [in5] -> M168/2(T1)
  [in6] -> M168/3(EB1)
  [in13] -> M168/4(CT3)
  [in17] -> M168/5(T3)
  [in18] -> M168/6(EB3)
  M168/1(LL1) -> Eval167/1(In1)
  M168/2(LL3) -> Eval167/2(In3)
  Eval167/1(Out1) -> To Workspace167/1
  [in1] -> M169/1(CT1)
  [in5] -> M169/2(T1)
  [in6] -> M169/3(EB1)
  [in13] -> M169/4(CT3)
  [in17] -> M169/5(T3)
  [in18] -> M169/6(EB3)
  M169/1(LL1) -> Eval168/1(In1)
  M169/2(LL3) -> Eval168/2(In3)
  Eval168/1(Out1) -> To Workspace168/1
  [in1] -> M170/1(CT1)
  [in5] -> M170/2(T1)
  [in6] -> M170/3(EB1)
  [in13] -> M170/4(CT3)
  [in17] -> M170/5(T3)
  [in18] -> M170/6(EB3)
  M170/1(LL1) -> Eval169/1(In1)
  M170/2(LL3) -> Eval169/2(In3)
  Eval169/1(Out1) -> To Workspace169/1
  [in1] -> M171/1(CT1)
  [in5] -> M171/2(T1)
  [in6] -> M171/3(EB1)
  [in13] -> M171/4(CT3)
  [in17] -> M171/5(T3)
  [in18] -> M171/6(EB3)
  M171/1(LL1) -> Eval170/1(In1)
  M171/2(LL3) -> Eval170/2(In3)
  Eval170/1(Out1) -> To Workspace170/1
  [in1] -> M172/1(CT1)
  [in5] -> M172/2(T1)
  [in6] -> M172/3(EB1)
  [in13] -> M172/4(CT3)
  [in17] -> M172/5(T3)
  [in18] -> M172/6(EB3)
  M172/1(LL1) -> Eval171/1(In1)
  M172/2(LL3) -> Eval171/2(In3)
  Eval171/1(Out1) -> To Workspace171/1
  [in1] -> M173/1(CT1)
  [in5] -> M173/2(T1)
  [in6] -> M173/3(EB1)
  [in13] -> M173/4(CT3)
  [in17] -> M173/5(T3)
  [in18] -> M173/6(EB3)
  M173/1(LL1) -> Eval172/1(In1)
  M173/2(LL3) -> Eval172/2(In3)
  Eval172/1(Out1) -> To Workspace172/1
  [in1] -> M174/1(CT1)
  [in5] -> M174/2(T1)
  [in6] -> M174/3(EB1)
  [in13] -> M174/4(CT3)
  [in17] -> M174/5(T3)
  [in18] -> M174/6(EB3)
  M174/1(LL1) -> Eval173/1(In1)
  M174/2(LL3) -> Eval173/2(In3)
  Eval173/1(Out1) -> To Workspace173/1
  [in1] -> M175/1(CT1)
  [in5] -> M175/2(T1)
  [in6] -> M175/3(EB1)
  [in13] -> M175/4(CT3)
  [in17] -> M175/5(T3)
  [in18] -> M175/6(EB3)
  M175/1(LL1) -> Eval174/1(In1)
  M175/2(LL3) -> Eval174/2(In3)
  Eval174/1(Out1) -> To Workspace174/1
  [in1] -> M176/1(CT1)
  [in5] -> M176/2(T1)
  [in6] -> M176/3(EB1)
  [in13] -> M176/4(CT3)
  [in17] -> M176/5(T3)
  [in18] -> M176/6(EB3)
  M176/1(LL1) -> Eval175/1(In1)
  M176/2(LL3) -> Eval175/2(In3)
  Eval175/1(Out1) -> To Workspace175/1
  [in1] -> M177/1(CT1)
  [in5] -> M177/2(T1)
  [in6] -> M177/3(EB1)
  [in13] -> M177/4(CT3)
  [in17] -> M177/5(T3)
  [in18] -> M177/6(EB3)
  M177/1(LL1) -> Eval176/1(In1)
  M177/2(LL3) -> Eval176/2(In3)
  Eval176/1(Out1) -> To Workspace176/1
  [in1] -> M178/1(CT1)
  [in5] -> M178/2(T1)
  [in6] -> M178/3(EB1)
  [in13] -> M178/4(CT3)
  [in17] -> M178/5(T3)
  [in18] -> M178/6(EB3)
  M178/1(LL1) -> Eval177/1(In1)
  M178/2(LL3) -> Eval177/2(In3)
  Eval177/1(Out1) -> To Workspace177/1
  [in1] -> M179/1(CT1)
  [in5] -> M179/2(T1)
  [in6] -> M179/3(EB1)
  [in13] -> M179/4(CT3)
  [in17] -> M179/5(T3)
  [in18] -> M179/6(EB3)
  M179/1(LL1) -> Eval178/1(In1)
  M179/2(LL3) -> Eval178/2(In3)
  Eval178/1(Out1) -> To Workspace178/1
  [in1] -> M180/1(CT1)
  [in5] -> M180/2(T1)
  [in6] -> M180/3(EB1)
  [in13] -> M180/4(CT3)
  [in17] -> M180/5(T3)
  [in18] -> M180/6(EB3)
  M180/1(LL1) -> Eval179/1(In1)
  M180/2(LL3) -> Eval179/2(In3)
  Eval179/1(Out1) -> To Workspace179/1
  [in1] -> M181/1(CT1)
  [in5] -> M181/2(T1)
  [in6] -> M181/3(EB1)
  [in13] -> M181/4(CT3)
  [in17] -> M181/5(T3)
  [in18] -> M181/6(EB3)
  M181/1(LL1) -> Eval180/1(In1)
  M181/2(LL3) -> Eval180/2(In3)
  Eval180/1(Out1) -> To Workspace180/1
  [in1] -> M182/1(CT1)
  [in5] -> M182/2(T1)
  [in6] -> M182/3(EB1)
  [in13] -> M182/4(CT3)
  [in17] -> M182/5(T3)
  [in18] -> M182/6(EB3)
  M182/1(LL1) -> Eval181/1(In1)
  M182/2(LL3) -> Eval181/2(In3)
  Eval181/1(Out1) -> To Workspace181/1
  [in1] -> M183/1(CT1)
  [in5] -> M183/2(T1)
  [in6] -> M183/3(EB1)
  [in13] -> M183/4(CT3)
  [in17] -> M183/5(T3)
  [in18] -> M183/6(EB3)
  M183/1(LL1) -> Eval182/1(In1)
  M183/2(LL3) -> Eval182/2(In3)
  Eval182/1(Out1) -> To Workspace182/1
  [in1] -> M184/1(CT1)
  [in5] -> M184/2(T1)
  [in6] -> M184/3(EB1)
  [in13] -> M184/4(CT3)
  [in17] -> M184/5(T3)
  [in18] -> M184/6(EB3)
  M184/1(LL1) -> Eval183/1(In1)
  M184/2(LL3) -> Eval183/2(In3)
  Eval183/1(Out1) -> To Workspace183/1
  [in1] -> M185/1(CT1)
  [in5] -> M185/2(T1)
  [in6] -> M185/3(EB1)
  [in13] -> M185/4(CT3)
  [in17] -> M185/5(T3)
  [in18] -> M185/6(EB3)
  M185/1(LL1) -> Eval184/1(In1)
  M185/2(LL3) -> Eval184/2(In3)
  Eval184/1(Out1) -> To Workspace184/1
  [in1] -> M186/1(CT1)
  [in5] -> M186/2(T1)
  [in6] -> M186/3(EB1)
  [in13] -> M186/4(CT3)
  [in17] -> M186/5(T3)
  [in18] -> M186/6(EB3)
  M186/1(LL1) -> Eval185/1(In1)
  M186/2(LL3) -> Eval185/2(In3)
  Eval185/1(Out1) -> To Workspace185/1
  [in1] -> M187/1(CT1)
  [in5] -> M187/2(T1)
  [in6] -> M187/3(EB1)
  [in13] -> M187/4(CT3)
  [in17] -> M187/5(T3)
  [in18] -> M187/6(EB3)
  M187/1(LL1) -> Eval186/1(In1)
  M187/2(LL3) -> Eval186/2(In3)
  Eval186/1(Out1) -> To Workspace186/1
  [in1] -> M188/1(CT1)
  [in5] -> M188/2(T1)
  [in6] -> M188/3(EB1)
  [in13] -> M188/4(CT3)
  [in17] -> M188/5(T3)
  [in18] -> M188/6(EB3)
  M188/1(LL1) -> Eval187/1(In1)
  M188/2(LL3) -> Eval187/2(In3)
  Eval187/1(Out1) -> To Workspace187/1
  [in1] -> M189/1(CT1)
  [in5] -> M189/2(T1)
  [in6] -> M189/3(EB1)
  [in13] -> M189/4(CT3)
  [in17] -> M189/5(T3)
  [in18] -> M189/6(EB3)
  M189/1(LL1) -> Eval188/1(In1)
  M189/2(LL3) -> Eval188/2(In3)
  Eval188/1(Out1) -> To Workspace188/1
  [in1] -> M190/1(CT1)
  [in5] -> M190/2(T1)
  [in6] -> M190/3(EB1)
  [in13] -> M190/4(CT3)
  [in17] -> M190/5(T3)
  [in18] -> M190/6(EB3)
  M190/1(LL1) -> Eval189/1(In1)
  M190/2(LL3) -> Eval189/2(In3)
  Eval189/1(Out1) -> To Workspace189/1
  [in1] -> M191/1(CT1)
  [in5] -> M191/2(T1)
  [in6] -> M191/3(EB1)
  [in13] -> M191/4(CT3)
  [in17] -> M191/5(T3)
  [in18] -> M191/6(EB3)
  M191/1(LL1) -> Eval190/1(In1)
  M191/2(LL3) -> Eval190/2(In3)
  Eval190/1(Out1) -> To Workspace190/1
  [in1] -> M192/1(CT1)
  [in5] -> M192/2(T1)
  [in6] -> M192/3(EB1)
  [in13] -> M192/4(CT3)
  [in17] -> M192/5(T3)
  [in18] -> M192/6(EB3)
  M192/1(LL1) -> Eval191/1(In1)
  M192/2(LL3) -> Eval191/2(In3)
  Eval191/1(Out1) -> To Workspace191/1
  [in1] -> M193/1(CT1)
  [in5] -> M193/2(T1)
  [in6] -> M193/3(EB1)
  [in13] -> M193/4(CT3)
  [in17] -> M193/5(T3)
  [in18] -> M193/6(EB3)
  M193/1(LL1) -> Eval192/1(In1)
  M193/2(LL3) -> Eval192/2(In3)
  Eval192/1(Out1) -> To Workspace192/1
  [in1] -> M194/1(CT1)
  [in5] -> M194/2(T1)
  [in6] -> M194/3(EB1)
  [in13] -> M194/4(CT3)
  [in17] -> M194/5(T3)
  [in18] -> M194/6(EB3)
  M194/1(LL1) -> Eval193/1(In1)
  M194/2(LL3) -> Eval193/2(In3)
  Eval193/1(Out1) -> To Workspace193/1
  [in1] -> M195/1(CT1)
  [in5] -> M195/2(T1)
  [in6] -> M195/3(EB1)
  [in13] -> M195/4(CT3)
  [in17] -> M195/5(T3)
  [in18] -> M195/6(EB3)
  M195/1(LL1) -> Eval194/1(In1)
  M195/2(LL3) -> Eval194/2(In3)
  Eval194/1(Out1) -> To Workspace194/1
  [in1] -> M196/1(CT1)
  [in5] -> M196/2(T1)
  [in6] -> M196/3(EB1)
  [in13] -> M196/4(CT3)
  [in17] -> M196/5(T3)
  [in18] -> M196/6(EB3)
  M196/1(LL1) -> Eval195/1(In1)
  M196/2(LL3) -> Eval195/2(In3)
  Eval195/1(Out1) -> To Workspace195/1
  [in1] -> M197/1(CT1)
  [in5] -> M197/2(T1)
  [in6] -> M197/3(EB1)
  [in13] -> M197/4(CT3)
  [in17] -> M197/5(T3)
  [in18] -> M197/6(EB3)
  M197/1(LL1) -> Eval196/1(In1)
  M197/2(LL3) -> Eval196/2(In3)
  Eval196/1(Out1) -> To Workspace196/1
  [in1] -> M198/1(CT1)
  [in5] -> M198/2(T1)
  [in6] -> M198/3(EB1)
  [in13] -> M198/4(CT3)
  [in17] -> M198/5(T3)
  [in18] -> M198/6(EB3)
  M198/1(LL1) -> Eval197/1(In1)
  M198/2(LL3) -> Eval197/2(In3)
  Eval197/1(Out1) -> To Workspace197/1
  [in1] -> M199/1(CT1)
  [in5] -> M199/2(T1)
  [in6] -> M199/3(EB1)
  [in13] -> M199/4(CT3)
  [in17] -> M199/5(T3)
  [in18] -> M199/6(EB3)
  M199/1(LL1) -> Eval198/1(In1)
  M199/2(LL3) -> Eval198/2(In3)
  Eval198/1(Out1) -> To Workspace198/1
  [in1] -> M221/1(CT1)
  [in5] -> M221/2(T1)
  [in6] -> M221/3(EB1)
  [in13] -> M221/4(CT3)
  [in17] -> M221/5(T3)
  [in18] -> M221/6(EB3)
  M221/1(LL1) -> Eval220/1(In1)
  M221/2(LL3) -> Eval220/2(In3)
  Eval220/1(Out1) -> To Workspace220/1
  [in1] -> M222/1(CT1)
  [in5] -> M222/2(T1)
  [in6] -> M222/3(EB1)
  [in13] -> M222/4(CT3)
  [in17] -> M222/5(T3)
  [in18] -> M222/6(EB3)
  M222/1(LL1) -> Eval221/1(In1)
  M222/2(LL3) -> Eval221/2(In3)
  Eval221/1(Out1) -> To Workspace221/1
  [in1] -> M223/1(CT1)
  [in5] -> M223/2(T1)
  [in6] -> M223/3(EB1)
  [in13] -> M223/4(CT3)
  [in17] -> M223/5(T3)
  [in18] -> M223/6(EB3)
  M223/1(LL1) -> Eval222/1(In1)
  M223/2(LL3) -> Eval222/2(In3)
  Eval222/1(Out1) -> To Workspace222/1
  [in1] -> M224/1(CT1)
  [in5] -> M224/2(T1)
  [in6] -> M224/3(EB1)
  [in13] -> M224/4(CT3)
  [in17] -> M224/5(T3)
  [in18] -> M224/6(EB3)
  M224/1(LL1) -> Eval223/1(In1)
  M224/2(LL3) -> Eval223/2(In3)
  Eval223/1(Out1) -> To Workspace223/1
  [in1] -> M225/1(CT1)
  [in5] -> M225/2(T1)
  [in6] -> M225/3(EB1)
  [in13] -> M225/4(CT3)
  [in17] -> M225/5(T3)
  [in18] -> M225/6(EB3)
  M225/1(LL1) -> Eval224/1(In1)
  M225/2(LL3) -> Eval224/2(In3)
  Eval224/1(Out1) -> To Workspace224/1
  [in1] -> M226/1(CT1)
  [in5] -> M226/2(T1)
  [in6] -> M226/3(EB1)
  [in13] -> M226/4(CT3)
  [in17] -> M226/5(T3)
  [in18] -> M226/6(EB3)
  M226/1(LL1) -> Eval225/1(In1)
  M226/2(LL3) -> Eval225/2(In3)
  Eval225/1(Out1) -> To Workspace225/1
  [in1] -> M227/1(CT1)
  [in5] -> M227/2(T1)
  [in6] -> M227/3(EB1)
  [in13] -> M227/4(CT3)
  [in17] -> M227/5(T3)
  [in18] -> M227/6(EB3)
  M227/1(LL1) -> Eval226/1(In1)
  M227/2(LL3) -> Eval226/2(In3)
  Eval226/1(Out1) -> To Workspace226/1
  [in1] -> M228/1(CT1)
  [in5] -> M228/2(T1)
  [in6] -> M228/3(EB1)
  [in13] -> M228/4(CT3)
  [in17] -> M228/5(T3)
  [in18] -> M228/6(EB3)
  M228/1(LL1) -> Eval227/1(In1)
  M228/2(LL3) -> Eval227/2(In3)
  Eval227/1(Out1) -> To Workspace227/1
  [in1] -> M229/1(CT1)
  [in5] -> M229/2(T1)
  [in6] -> M229/3(EB1)
  [in13] -> M229/4(CT3)
  [in17] -> M229/5(T3)
  [in18] -> M229/6(EB3)
  M229/1(LL1) -> Eval228/1(In1)
  M229/2(LL3) -> Eval228/2(In3)
  Eval228/1(Out1) -> To Workspace228/1
  [in1] -> M230/1(CT1)
  [in5] -> M230/2(T1)
  [in6] -> M230/3(EB1)
  [in13] -> M230/4(CT3)
  [in17] -> M230/5(T3)
  [in18] -> M230/6(EB3)
  M230/1(LL1) -> Eval229/1(In1)
  M230/2(LL3) -> Eval229/2(In3)
  Eval229/1(Out1) -> To Workspace229/1
  [in1] -> M231/1(CT1)
  [in5] -> M231/2(T1)
  [in6] -> M231/3(EB1)
  [in13] -> M231/4(CT3)
  [in17] -> M231/5(T3)
  [in18] -> M231/6(EB3)
  M231/1(LL1) -> Eval230/1(In1)
  M231/2(LL3) -> Eval230/2(In3)
  Eval230/1(Out1) -> To Workspace230/1
  [in1] -> M232/1(CT1)
  [in5] -> M232/2(T1)
  [in6] -> M232/3(EB1)
  [in13] -> M232/4(CT3)
  [in17] -> M232/5(T3)
  [in18] -> M232/6(EB3)
  M232/1(LL1) -> Eval231/1(In1)
  M232/2(LL3) -> Eval231/2(In3)
  Eval231/1(Out1) -> To Workspace231/1
  [in1] -> M233/1(CT1)
  [in5] -> M233/2(T1)
  [in6] -> M233/3(EB1)
  [in13] -> M233/4(CT3)
  [in17] -> M233/5(T3)
  [in18] -> M233/6(EB3)
  M233/1(LL1) -> Eval232/1(In1)
  M233/2(LL3) -> Eval232/2(In3)
  Eval232/1(Out1) -> To Workspace232/1
  [in1] -> M234/1(CT1)
  [in5] -> M234/2(T1)
  [in6] -> M234/3(EB1)
  [in13] -> M234/4(CT3)
  [in17] -> M234/5(T3)
  [in18] -> M234/6(EB3)
  M234/1(LL1) -> Eval233/1(In1)
  M234/2(LL3) -> Eval233/2(In3)
  Eval233/1(Out1) -> To Workspace233/1
  [in1] -> M235/1(CT1)
  [in5] -> M235/2(T1)
  [in6] -> M235/3(EB1)
  [in13] -> M235/4(CT3)
  [in17] -> M235/5(T3)
  [in18] -> M235/6(EB3)
  M235/1(LL1) -> Eval234/1(In1)
  M235/2(LL3) -> Eval234/2(In3)
  Eval234/1(Out1) -> To Workspace234/1
  [in1] -> M236/1(CT1)
  [in5] -> M236/2(T1)
  [in6] -> M236/3(EB1)
  [in13] -> M236/4(CT3)
  [in17] -> M236/5(T3)
  [in18] -> M236/6(EB3)
  M236/1(LL1) -> Eval235/1(In1)
  M236/2(LL3) -> Eval235/2(In3)
  Eval235/1(Out1) -> To Workspace235/1
  [in1] -> M237/1(CT1)
  [in5] -> M237/2(T1)
  [in6] -> M237/3(EB1)
  [in13] -> M237/4(CT3)
  [in17] -> M237/5(T3)
  [in18] -> M237/6(EB3)
  M237/1(LL1) -> Eval236/1(In1)
  M237/2(LL3) -> Eval236/2(In3)
  Eval236/1(Out1) -> To Workspace236/1
  [in1] -> M238/1(CT1)
  [in5] -> M238/2(T1)
  [in6] -> M238/3(EB1)
  [in13] -> M238/4(CT3)
  [in17] -> M238/5(T3)
  [in18] -> M238/6(EB3)
  M238/1(LL1) -> Eval237/1(In1)
  M238/2(LL3) -> Eval237/2(In3)
  Eval237/1(Out1) -> To Workspace237/1
  [in1] -> M239/1(CT1)
  [in5] -> M239/2(T1)
  [in6] -> M239/3(EB1)
  [in13] -> M239/4(CT3)
  [in17] -> M239/5(T3)
  [in18] -> M239/6(EB3)
  M239/1(LL1) -> Eval238/1(In1)
  M239/2(LL3) -> Eval238/2(In3)
  Eval238/1(Out1) -> To Workspace238/1
  [in1] -> M240/1(CT1)
  [in5] -> M240/2(T1)
  [in6] -> M240/3(EB1)
  [in13] -> M240/4(CT3)
  [in17] -> M240/5(T3)
  [in18] -> M240/6(EB3)
  M240/1(LL1) -> Eval239/1(In1)
  M240/2(LL3) -> Eval239/2(In3)
  Eval239/1(Out1) -> To Workspace239/1
  [in1] -> M241/1(CT1)
  [in5] -> M241/2(T1)
  [in6] -> M241/3(EB1)
  [in13] -> M241/4(CT3)
  [in17] -> M241/5(T3)
  [in18] -> M241/6(EB3)
  M241/1(LL1) -> Eval240/1(In1)
  M241/2(LL3) -> Eval240/2(In3)
  Eval240/1(Out1) -> To Workspace240/1
  [in1] -> M242/1(CT1)
  [in5] -> M242/2(T1)
  [in6] -> M242/3(EB1)
  [in13] -> M242/4(CT3)
  [in17] -> M242/5(T3)
  [in18] -> M242/6(EB3)
  M242/1(LL1) -> Eval241/1(In1)
  M242/2(LL3) -> Eval241/2(In3)
  Eval241/1(Out1) -> To Workspace241/1
  [in1] -> M243/1(CT1)
  [in5] -> M243/2(T1)
  [in6] -> M243/3(EB1)
  [in13] -> M243/4(CT3)
  [in17] -> M243/5(T3)
  [in18] -> M243/6(EB3)
  M243/1(LL1) -> Eval242/1(In1)
  M243/2(LL3) -> Eval242/2(In3)
  Eval242/1(Out1) -> To Workspace242/1
  [in1] -> M244/1(CT1)
  [in5] -> M244/2(T1)
  [in6] -> M244/3(EB1)
  [in13] -> M244/4(CT3)
  [in17] -> M244/5(T3)
  [in18] -> M244/6(EB3)
  M244/1(LL1) -> Eval243/1(In1)
  M244/2(LL3) -> Eval243/2(In3)
  Eval243/1(Out1) -> To Workspace243/1
  [in1] -> M245/1(CT1)
  [in5] -> M245/2(T1)
  [in6] -> M245/3(EB1)
  [in13] -> M245/4(CT3)
  [in17] -> M245/5(T3)
  [in18] -> M245/6(EB3)
  M245/1(LL1) -> Eval244/1(In1)
  M245/2(LL3) -> Eval244/2(In3)
  Eval244/1(Out1) -> To Workspace244/1
  [in1] -> M246/1(CT1)
  [in5] -> M246/2(T1)
  [in6] -> M246/3(EB1)
  [in13] -> M246/4(CT3)
  [in17] -> M246/5(T3)
  [in18] -> M246/6(EB3)
  M246/1(LL1) -> Eval245/1(In1)
  M246/2(LL3) -> Eval245/2(In3)
  Eval245/1(Out1) -> To Workspace245/1
  Inputs/1(CT1) -> dtc_CT1/1
  dtc_CT1/1 -> CPSUT/1(CT1), [in1]
  Inputs/2(T1) -> dtc_T1/1
  dtc_T1/1 -> CPSUT/2(T1), [in5]
  Inputs/3(EB1) -> dtc_EB1/1
  dtc_EB1/1 -> CPSUT/3(EB1), [in6]
  Inputs/4(CT3) -> dtc_CT3/1
  dtc_CT3/1 -> CPSUT/4(CT3), [in13]
  Inputs/5(T3) -> dtc_T3/1
  dtc_T3/1 -> CPSUT/5(T3), [in17]
  Inputs/6(EB3) -> dtc_EB3/1
  dtc_EB3/1 -> CPSUT/6(EB3), [in18]

== system c00015M_harness/CPSUT ==
  note: VALUES
      | ---------------------------------
      | ControlType = 1 | 2 | 3
      | FillTank = 0 | 1
      | EmptyTank = 0 | 1
      | ManualReference between 0 and 1
      | Tempreature between 0 and 100
      | EmergencyButton = 0 | 1
      | LiquidLevel between 0 and 1 (hmax)
  note: Inputs For Tank2
  note: NAMES
      | --------------------------------------------
      | CT1 = ControlType Tank 1
      | F1 = Fill Tank 1
      | E1 = Empty Tank 1
      | MR1 = Manual Reference Tank1
      | T1 = Temperature Tank 1
      | EB1 = Emergency Button Tank 1
      | LL1 = Liquid Level 1
  note: Inputs For Tank3
  note: Inputs For Tank1
  CT1 : Inport
  T1 : Inport  Port=2
  EB1 : Inport  Port=3
  CT3 : Inport  Port=4
  T3 : Inport  Port=5
  EB3 : Inport  Port=6
  Tank1 : Subsystem
  Tank3 : Subsystem
  LL1 : Outport
  LL3 : Outport  Port=2
  wires:
  EB1/1 -> Tank1/3(EB1)
  Tank3/1(LL3) -> LL3/1, Tank1/4(LL3)
  T1/1 -> Tank1/2(T1)
  Tank1/1(LL1) -> LL1/1, Tank3/4(LL1)
  CT3/1 -> Tank3/1(CT3)
  EB3/1 -> Tank3/3(EB3)
  T3/1 -> Tank3/2(T3)
  CT1/1 -> Tank1/1(CT1)

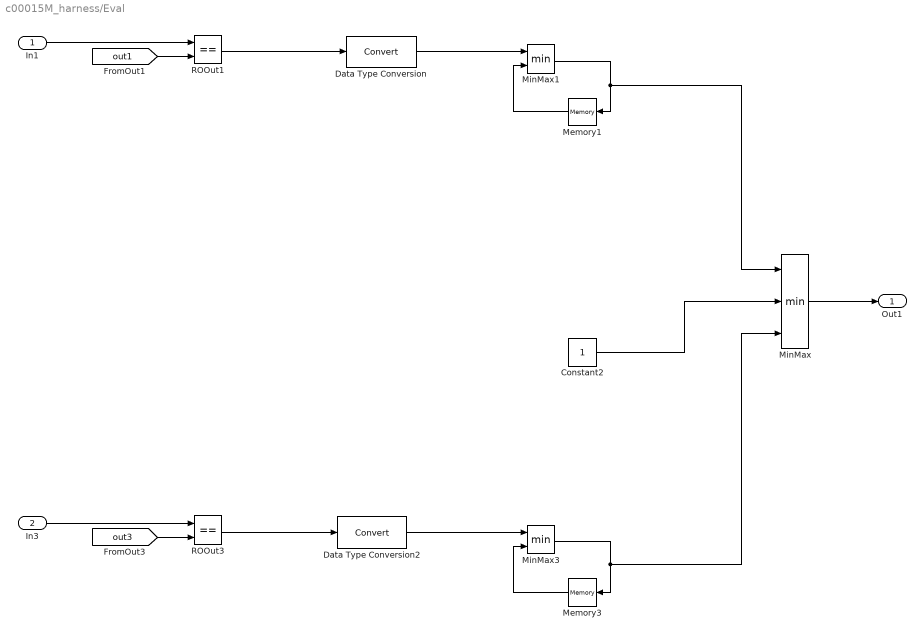
== system c00015M_harness/Eval ==
  In1 : Inport
  In3 : Inport  Port=2
  Constant2 : Constant
  Data Type Conversion : DataTypeConversion
  Data Type Conversion2 : DataTypeConversion
  Memory1 : Memory  InitialCondition=1
  Memory3 : Memory  InitialCondition=1
  MinMax : MinMax  Inputs=3
  MinMax1 : MinMax  Inputs=2
  MinMax3 : MinMax  Inputs=2
  ROOut1 : RelationalOperator  Operator===  OutDataTypeStr=boolean  RndMeth=Simplest
  ROOut3 : RelationalOperator  Operator===  OutDataTypeStr=boolean  RndMeth=Simplest
  Out1 : Outport
  wires:
  MinMax/1 -> Out1/1
  [out3] -> ROOut3/2
  In3/1 -> ROOut3/1
  [out1] -> ROOut1/2
  In1/1 -> ROOut1/1
  Memory1/1 -> MinMax1/2
  MinMax3/1 -> MinMax/3, Memory3/1
  ROOut3/1 -> Data Type Conversion2/1
  Memory3/1 -> MinMax3/2
  ROOut1/1 -> Data Type Conversion/1
  MinMax1/1 -> MinMax/1, Memory1/1
  Data Type Conversion/1 -> MinMax1/1
  Data Type Conversion2/1 -> MinMax3/1
  Constant2/1 -> MinMax/2

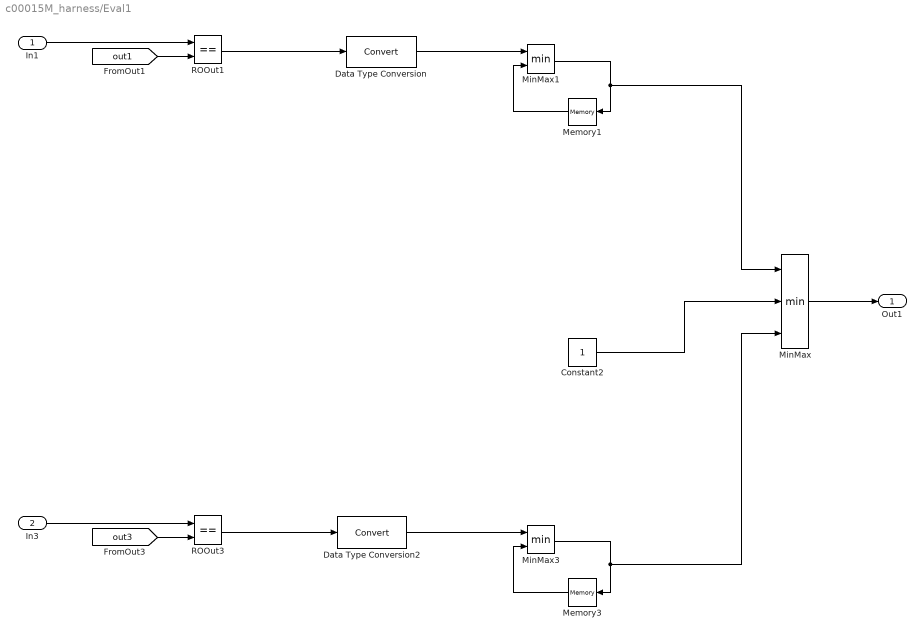
== system c00015M_harness/Eval1 ==
  In1 : Inport
  In3 : Inport  Port=2
  Constant2 : Constant
  Data Type Conversion : DataTypeConversion
  Data Type Conversion2 : DataTypeConversion
  Memory1 : Memory  InitialCondition=1
  Memory3 : Memory  InitialCondition=1
  MinMax : MinMax  Inputs=3
  MinMax1 : MinMax  Inputs=2
  MinMax3 : MinMax  Inputs=2
  ROOut1 : RelationalOperator  Operator===  OutDataTypeStr=boolean  RndMeth=Simplest
  ROOut3 : RelationalOperator  Operator===  OutDataTypeStr=boolean  RndMeth=Simplest
  Out1 : Outport
  wires:
  Data Type Conversion2/1 -> MinMax3/1
  Data Type Conversion/1 -> MinMax1/1
  MinMax1/1 -> Memory1/1, MinMax/1
  ROOut1/1 -> Data Type Conversion/1
  Memory3/1 -> MinMax3/2
  ROOut3/1 -> Data Type Conversion2/1
  MinMax3/1 -> Memory3/1, MinMax/3
  Memory1/1 -> MinMax1/2
  In1/1 -> ROOut1/1
  [out1] -> ROOut1/2
  In3/1 -> ROOut3/1
  [out3] -> ROOut3/2
  MinMax/1 -> Out1/1
  Constant2/1 -> MinMax/2
